simulink model "PID_Controller"  (Simulink 8.7)
settings: Solver=VariableStepAuto  StartTime=0.0  StopTime=10.0  RelTol=1e-3
values from neighbouring files (symbols this model uses):
  Fmatrix = [-1/sqrt(2) 0 1/sqrt(2) 1 ... (first row only)    [Inverse.m]
undefined symbols (not defined in the file or in its folder): Imatrix
libraries: dspmtrx3 x1
(part 1 of 3)
settings Model: Creator=as01398  LastModifiedBy=baideqian
settings DataIOCC: LimitDataPoints=off  SaveFormat=Dataset  OutputOption=SpecifiedOutputTimes  OutputTimes=[0:0.2:10]
settings DebuggingCC: UnderspecifiedInitializationDetection=Simplified  MergeDetectMultiDrivingBlocksExec=error
settings HardwareCC: ProdBitPerPointer=64  ProdLargestAtomicFloat=Float  ProdIntDivRoundTo=Zero  ProdEndianess=LittleEndian  ProdWordSize=64  ProdHWDeviceType=Intel->x86-64 (Windows64)
settings ModelReferenceCC: PropagateSignalLabelsOutOfModel=on
settings ConfigComp: CovModelRefEnable=off

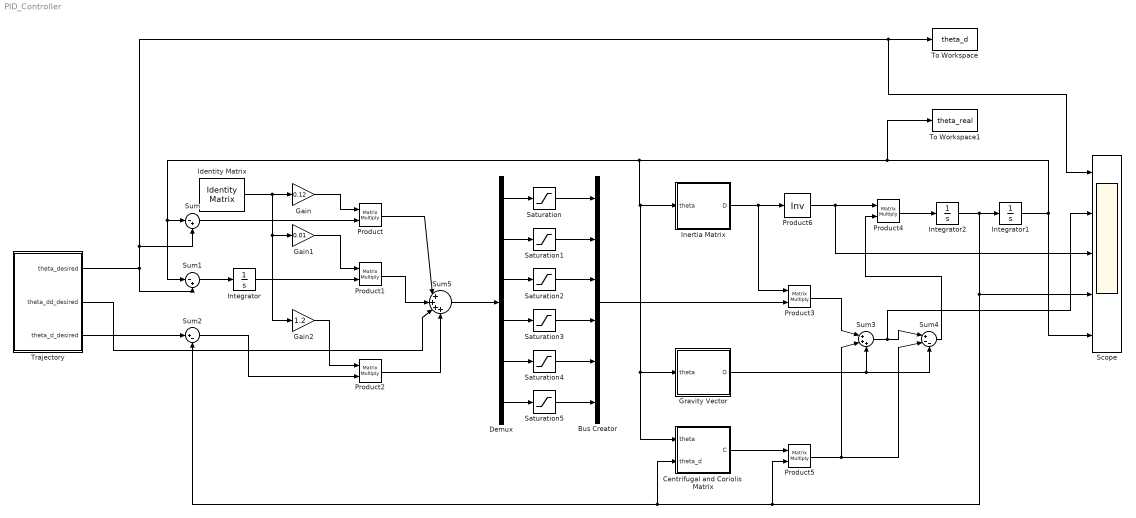
== system PID_Controller ==
  Bus Creator : BusCreator  Inputs=6
  Centrifugal and Coriolis  Matrix : Subsystem
  Demux : Demux  Outputs=6
  Gain : Gain  Gain=0.12
  Gain1 : Gain  Gain=0.01
  Gain2 : Gain  Gain=1.2
  Gravity Vector : Subsystem
  Identity Matrix : dspmtrx3/Identity Matrix  Inherit=off  N=6  Ts=1  dataType=double  isSigned=on  wordLen=16  udDataType=sfix(16)  fracBitsMode=Best precision  numFracBits=15  OutDataTypeStr=double  LastOutDataTypeStr=double
  Inertia Matrix : Subsystem
  Integrator : Integrator
  Integrator1 : Integrator
  Integrator2 : Integrator
  Product{,1..5} (6 alike) : Product  Multiplication=Matrix(*)
  Product6 : Product  Inputs=/  Multiplication=Matrix(*)
  Saturation : Saturate  UpperLimit=16  LowerLimit=-16
  Saturation1 : Saturate  UpperLimit=32  LowerLimit=-32
  Saturation2 : Saturate  UpperLimit=21  LowerLimit=-21
  Saturation3 : Saturate  UpperLimit=5  LowerLimit=-5
  Saturation4 : Saturate  UpperLimit=5  LowerLimit=-5
  Saturation5 : Saturate  UpperLimit=4  LowerLimit=-4
  Scope : Scope  NumInputPorts=5
  Sum : Sum  Inputs=|-+
  Sum1 : Sum  Inputs=|-+
  Sum2 : Sum  Inputs=|+-
  Sum3 : Sum  Inputs=|+++
  Sum4 : Sum  Inputs=|+--
  Sum5 : Sum  Inputs=|++++
  To Workspace : ToWorkspace  VariableName=theta_d  SampleTime=-1
  To Workspace1 : ToWorkspace  VariableName=theta_real  SampleTime=-1
  Trajectory : Subsystem
  wires:
  Trajectory/2(theta_dd_desired) -> Sum5/3
  Trajectory/1(theta_desired) -> Scope/1, To Workspace/1, Sum/2, Sum1/2
  Trajectory/3(theta_d_desired) -> Sum2/1
  Gain2/1 -> Product2/1
  Sum2/1 -> Product2/2
  Sum1/1 -> Integrator/1
  Integrator/1 -> Product1/2
  Gain1/1 -> Product1/1
  Identity Matrix/1 -> Gain2/1, Gain1/1, Gain/1
  Sum/1 -> Product/2
  Gain/1 -> Product/1
  Product2/1 -> Sum5/4
  Product1/1 -> Sum5/2
  Product/1 -> Sum5/1
  Sum5/1 -> Demux/1
  Demux/1 -> Saturation/1
  Demux/2 -> Saturation1/1
  Demux/3 -> Saturation2/1
  Demux/4 -> Saturation3/1
  Demux/5 -> Saturation4/1
  Demux/6 -> Saturation5/1
  Saturation/1 -> Bus Creator/1
  Saturation1/1 -> Bus Creator/2
  Saturation2/1 -> Bus Creator/3
  Saturation3/1 -> Bus Creator/4
  Saturation4/1 -> Bus Creator/5
  Saturation5/1 -> Bus Creator/6
  Inertia Matrix/1(D) -> Product6/1, Product3/1
  Product6/1 -> Scope/3, Product4/1
  Product4/1 -> Integrator2/1
  Centrifugal and Coriolis  Matrix/1(C) -> Product5/1
  Gravity Vector/1(G) -> Sum3/3, Sum4/3
  Product5/1 -> Sum4/2, Sum3/2
  Product3/1 -> Sum3/1
  Sum4/1 -> Product4/2
  Integrator2/1 -> Scope/4, Sum2/2, Centrifugal and Coriolis  Matrix/2(theta_d), Product5/2, Integrator1/1
  Integrator1/1 -> Scope/5, To Workspace1/1, Centrifugal and Coriolis  Matrix/1(theta), Gravity Vector/1(theta), Inertia Matrix/1(theta), Sum/1, Sum1/1
  Sum3/1 -> Scope/2, Sum4/1
  Bus Creator/1 -> Product3/2

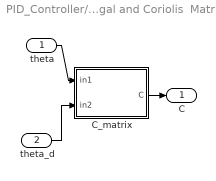
== system PID_Controller/Centrifugal and Coriolis  Matrix ==
  theta : Inport
  theta_d : Inport  Port=2
  C_matrix : MATLAB Function  TreatAsAtomicUnit=on
  C : Outport
  wires:
  theta_d/1 -> C_matrix/2(in2)
  theta/1 -> C_matrix/1(in1)
  C_matrix/1(C) -> C/1

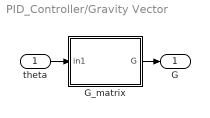
== system PID_Controller/Gravity Vector ==
  theta : Inport
  G_matrix : MATLAB Function  TreatAsAtomicUnit=on
  G : Outport
  wires:
  G_matrix/1(G) -> G/1
  theta/1 -> G_matrix/1(in1)

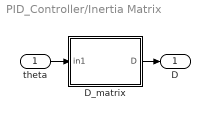
== system PID_Controller/Inertia Matrix ==
  theta : Inport
  D_matrix : MATLAB Function  TreatAsAtomicUnit=on
  D : Outport
  wires:
  D_matrix/1(D) -> D/1
  theta/1 -> D_matrix/1(in1)

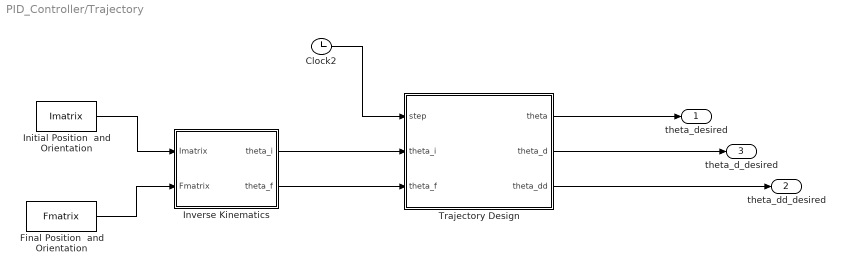
== system PID_Controller/Trajectory ==
  Clock2 : Clock
      settings: Decimation=1000
  Final Position  and Orientation : Constant  Value=Fmatrix
  Initial Position  and Orientation : Constant  Value=Imatrix
  Inverse Kinematics : MATLAB Function  TreatAsAtomicUnit=on
  Trajectory Design : MATLAB Function  TreatAsAtomicUnit=on
  theta_desired : Outport
  theta_dd_desired : Outport  Port=2
  theta_d_desired : Outport  Port=3
  wires:
  Trajectory Design/3(theta_dd) -> theta_dd_desired/1
  Trajectory Design/2(theta_d) -> theta_d_desired/1
  Trajectory Design/1(theta) -> theta_desired/1
  Inverse Kinematics/2(theta_f) -> Trajectory Design/3(theta_f)
  Inverse Kinematics/1(theta_i) -> Trajectory Design/2(theta_i)
  Final Position  and Orientation/1 -> Inverse Kinematics/2(Fmatrix)
  Initial Position  and Orientation/1 -> Inverse Kinematics/1(Imatrix)
  Clock2/1 -> Trajectory Design/1(step)
